simulink model "wiggler_frf_adxl"  (R2018a)
settings: Solver=FixedStepDiscrete  StartTime=0.0  StopTime=10.0  RelTol=1e-3
PreLoadFcn:
  | waijung.modelPreload; % Required for working with Waijung Blockset. Do not remove.
undefined symbols (not defined in the file or in its folder): HSEOSC, Link, LQFP144, ST, STM32F446ZE
libraries: commsynccomp2 x38, simulink x10, stm32f4_io_lib x3, dspstat3 x2, stm32f4_device_config_lib x1, dspbuff3 x1
(part 2 of 4)

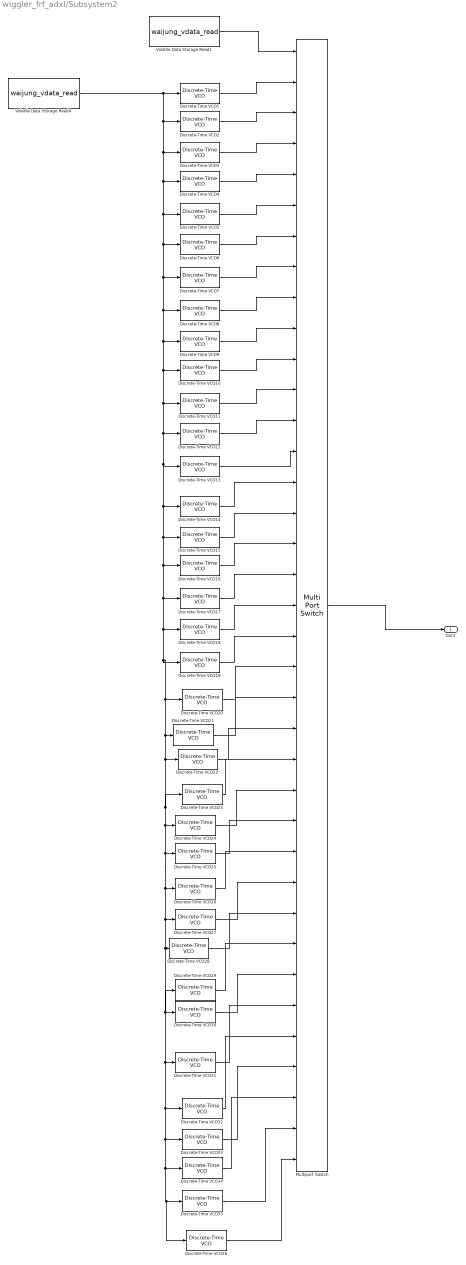
== system wiggler_frf_adxl/Subsystem2 ==
  Discrete-Time VCO1 : commsynccomp2/Discrete-Time VCO  Ac=1  Fc=0  Kc=1  Ph=0  ts=1e-3
      settings: SourceProductName=Communications System Toolbox  SourceProductBaseCode=CM
  Discrete-Time VCO10 : commsynccomp2/Discrete-Time VCO  Ac=1  Fc=0  Kc=1  Ph=(90/180)*pi  ts=1e-3
      settings: SourceProductName=Communications System Toolbox  SourceProductBaseCode=CM
  Discrete-Time VCO11 : commsynccomp2/Discrete-Time VCO  Ac=1  Fc=0  Kc=1  Ph=(100/180)*pi  ts=1e-3
      settings: SourceProductName=Communications System Toolbox  SourceProductBaseCode=CM
  Discrete-Time VCO12 : commsynccomp2/Discrete-Time VCO  Ac=1  Fc=0  Kc=1  Ph=(110/180)*pi  ts=1e-3
      settings: SourceProductName=Communications System Toolbox  SourceProductBaseCode=CM
  Discrete-Time VCO13 : commsynccomp2/Discrete-Time VCO  Ac=1  Fc=0  Kc=1  Ph=(120/180)*pi  ts=1e-3
      settings: SourceProductName=Communications System Toolbox  SourceProductBaseCode=CM
  Discrete-Time VCO14 : commsynccomp2/Discrete-Time VCO  Ac=1  Fc=0  Kc=1  Ph=(130/180)*pi  ts=1e-3
      settings: SourceProductName=Communications System Toolbox  SourceProductBaseCode=CM
  Discrete-Time VCO15 : commsynccomp2/Discrete-Time VCO  Ac=1  Fc=0  Kc=1  Ph=(140/180)*pi  ts=1e-3
      settings: SourceProductName=Communications System Toolbox  SourceProductBaseCode=CM
  Discrete-Time VCO16 : commsynccomp2/Discrete-Time VCO  Ac=1  Fc=0  Kc=1  Ph=(150/180)*pi  ts=1e-3
      settings: SourceProductName=Communications System Toolbox  SourceProductBaseCode=CM
  Discrete-Time VCO17 : commsynccomp2/Discrete-Time VCO  Ac=1  Fc=0  Kc=1  Ph=(160/180)*pi  ts=1e-3
      settings: SourceProductName=Communications System Toolbox  SourceProductBaseCode=CM
  Discrete-Time VCO18 : commsynccomp2/Discrete-Time VCO  Ac=1  Fc=0  Kc=1  Ph=(170/180)*pi  ts=1e-3
      settings: SourceProductName=Communications System Toolbox  SourceProductBaseCode=CM
  Discrete-Time VCO19 : commsynccomp2/Discrete-Time VCO  Ac=1  Fc=0  Kc=1  Ph=(180/180)*pi  ts=1e-3
      settings: SourceProductName=Communications System Toolbox  SourceProductBaseCode=CM
  Discrete-Time VCO2 : commsynccomp2/Discrete-Time VCO  Ac=1  Fc=0  Kc=1  Ph=(10/180)*pi  ts=1e-3
      settings: SourceProductName=Communications System Toolbox  SourceProductBaseCode=CM
  Discrete-Time VCO20 : commsynccomp2/Discrete-Time VCO  Ac=1  Fc=0  Kc=1  Ph=(190/180)*pi  ts=1e-3
      settings: SourceProductName=Communications System Toolbox  SourceProductBaseCode=CM
  Discrete-Time VCO21 : commsynccomp2/Discrete-Time VCO  Ac=1  Fc=0  Kc=1  Ph=(200/180)*pi  ts=1e-3
      settings: SourceProductName=Communications System Toolbox  SourceProductBaseCode=CM
  Discrete-Time VCO22 : commsynccomp2/Discrete-Time VCO  Ac=1  Fc=0  Kc=1  Ph=(210/180)*pi  ts=1e-3
      settings: SourceProductName=Communications System Toolbox  SourceProductBaseCode=CM
  Discrete-Time VCO23 : commsynccomp2/Discrete-Time VCO  Ac=1  Fc=0  Kc=1  Ph=(220/180)*pi  ts=1e-3
      settings: SourceProductName=Communications System Toolbox  SourceProductBaseCode=CM
  Discrete-Time VCO24 : commsynccomp2/Discrete-Time VCO  Ac=1  Fc=0  Kc=1  Ph=(230/180)*pi  ts=1e-3
      settings: SourceProductName=Communications System Toolbox  SourceProductBaseCode=CM
  Discrete-Time VCO25 : commsynccomp2/Discrete-Time VCO  Ac=1  Fc=0  Kc=1  Ph=(240/180)*pi  ts=1e-3
      settings: SourceProductName=Communications System Toolbox  SourceProductBaseCode=CM
  Discrete-Time VCO26 : commsynccomp2/Discrete-Time VCO  Ac=1  Fc=0  Kc=1  Ph=(250/180)*pi  ts=1e-3
      settings: SourceProductName=Communications System Toolbox  SourceProductBaseCode=CM
  Discrete-Time VCO27 : commsynccomp2/Discrete-Time VCO  Ac=1  Fc=0  Kc=1  Ph=(260/180)*pi  ts=1e-3
      settings: SourceProductName=Communications System Toolbox  SourceProductBaseCode=CM
  Discrete-Time VCO28 : commsynccomp2/Discrete-Time VCO  Ac=1  Fc=0  Kc=1  Ph=(270/180)*pi  ts=1e-3
      settings: SourceProductName=Communications System Toolbox  SourceProductBaseCode=CM
  Discrete-Time VCO29 : commsynccomp2/Discrete-Time VCO  Ac=1  Fc=0  Kc=1  Ph=(280/180)*pi  ts=1e-3
      settings: SourceProductName=Communications System Toolbox  SourceProductBaseCode=CM
  Discrete-Time VCO3 : commsynccomp2/Discrete-Time VCO  Ac=1  Fc=0  Kc=1  Ph=(20/180)*pi  ts=1e-3
      settings: SourceProductName=Communications System Toolbox  SourceProductBaseCode=CM
  Discrete-Time VCO30 : commsynccomp2/Discrete-Time VCO  Ac=1  Fc=0  Kc=1  Ph=(290/180)*pi  ts=1e-3
      settings: SourceProductName=Communications System Toolbox  SourceProductBaseCode=CM
  Discrete-Time VCO31 : commsynccomp2/Discrete-Time VCO  Ac=1  Fc=0  Kc=1  Ph=(300/180)*pi  ts=1e-3
      settings: SourceProductName=Communications System Toolbox  SourceProductBaseCode=CM
  Discrete-Time VCO32 : commsynccomp2/Discrete-Time VCO  Ac=1  Fc=0  Kc=1  Ph=(310/180)*pi  ts=1e-3
      settings: SourceProductName=Communications System Toolbox  SourceProductBaseCode=CM
  Discrete-Time VCO33 : commsynccomp2/Discrete-Time VCO  Ac=1  Fc=0  Kc=1  Ph=(320/180)*pi  ts=1e-3
      settings: SourceProductName=Communications System Toolbox  SourceProductBaseCode=CM
  Discrete-Time VCO34 : commsynccomp2/Discrete-Time VCO  Ac=1  Fc=0  Kc=1  Ph=(330/180)*pi  ts=1e-3
      settings: SourceProductName=Communications System Toolbox  SourceProductBaseCode=CM
  Discrete-Time VCO35 : commsynccomp2/Discrete-Time VCO  Ac=1  Fc=0  Kc=1  Ph=(340/180)*pi  ts=1e-3
      settings: SourceProductName=Communications System Toolbox  SourceProductBaseCode=CM
  Discrete-Time VCO36 : commsynccomp2/Discrete-Time VCO  Ac=1  Fc=0  Kc=1  Ph=(350/180)*pi  ts=1e-3
      settings: SourceProductName=Communications System Toolbox  SourceProductBaseCode=CM
  Discrete-Time VCO4 : commsynccomp2/Discrete-Time VCO  Ac=1  Fc=0  Kc=1  Ph=(30/180)*pi  ts=1e-3
      settings: SourceProductName=Communications System Toolbox  SourceProductBaseCode=CM
  Discrete-Time VCO5 : commsynccomp2/Discrete-Time VCO  Ac=1  Fc=0  Kc=1  Ph=(40/180)*pi  ts=1e-3
      settings: SourceProductName=Communications System Toolbox  SourceProductBaseCode=CM
  Discrete-Time VCO6 : commsynccomp2/Discrete-Time VCO  Ac=1  Fc=0  Kc=1  Ph=(50/180)*pi  ts=1e-3
      settings: SourceProductName=Communications System Toolbox  SourceProductBaseCode=CM
  Discrete-Time VCO7 : commsynccomp2/Discrete-Time VCO  Ac=1  Fc=0  Kc=1  Ph=(60/180)*pi  ts=1e-3
      settings: SourceProductName=Communications System Toolbox  SourceProductBaseCode=CM
  Discrete-Time VCO8 : commsynccomp2/Discrete-Time VCO  Ac=1  Fc=0  Kc=1  Ph=(70/180)*pi  ts=1e-3
      settings: SourceProductName=Communications System Toolbox  SourceProductBaseCode=CM
  Discrete-Time VCO9 : commsynccomp2/Discrete-Time VCO  Ac=1  Fc=0  Kc=1  Ph=(80/180)*pi  ts=1e-3
      settings: SourceProductName=Communications System Toolbox  SourceProductBaseCode=CM
  Multiport Switch : MultiPortSwitch  DataPortOrder=Zero-based contiguous  Inputs=36  zeroidx=on
  Volatile Data Storage Read1 : S-Function  FunctionName=waijung_vdata_read  Parameters=storagename,varname,sampletime,sampletimestr,blockid,storagetype,storagetypestr  SFunctionDeploymentMode=off  EnableBusSupport=off  mask(waijung_vdata_read){storagename=Phase, varname=VolatileDataStorage7_Phase, sampletime=.001, sampletimestr=-1, blockid=Subsystem2VolatileDataStorageRead1, storagetype=double, storagetypestr=double}
      mask prompts: storagename "Storage Name"; varname "Variable name"; sampletime "Sample time (sec)"; sampletimestr "Compiled sample time (sec) in string"; storagetype "Data type"; storagetypestr "Data type string"
      mask help: This block implements read data from a buffer.
      mask init:
      | waijung_vdata_read_callback('init');
      mask Help: web(fullfile(waijungdocroot,'Volatile_Data_Storage_Read.htm'))
      mask TypeOptions storagename: Laser | Ax | flag | fx | fy | Ay | Phase
      mask Callback storagename: waijung_vdata_read_callback('storagename');
      mask Callback varname: waijung_vdata_read_callback('varname');
      mask Callback sampletime: waijung_vdata_read_callback('sampletime');
      mask Callback sampletimestr: waijung_vdata_read_callback('sampletimestr');
      mask Callback blockid: waijung_vdata_read_callback('blockid');
      mask Callback storagetype: waijung_vdata_read_callback('storagetype');
      mask Display: text(0.05, 0.5, 'Buffer: Phase','ver','middle','hor','left');port_label('output',1,'D1(double)')
  Volatile Data Storage Read4 : S-Function  FunctionName=waijung_vdata_read  Parameters=storagename,varname,sampletime,sampletimestr,blockid,storagetype,storagetypestr  SFunctionDeploymentMode=off  EnableBusSupport=off  mask(waijung_vdata_read){storagename=fy, varname=VolatileDataStorage5_fy, sampletime=.001, sampletimestr=-1, blockid=Subsystem2VolatileDataStorageRead4, storagetype=double, storagetypestr=double}
      mask prompts: storagename "Storage Name"; varname "Variable name"; sampletime "Sample time (sec)"; sampletimestr "Compiled sample time (sec) in string"; storagetype "Data type"; storagetypestr "Data type string"
      mask help: This block implements read data from a buffer.
      mask init:
      | waijung_vdata_read_callback('init');
      mask Help: web(fullfile(waijungdocroot,'Volatile_Data_Storage_Read.htm'))
      mask TypeOptions storagename: Laser | Ax | flag | fx | fy | Ay | Phase
      mask Callback storagename: waijung_vdata_read_callback('storagename');
      mask Callback varname: waijung_vdata_read_callback('varname');
      mask Callback sampletime: waijung_vdata_read_callback('sampletime');
      mask Callback sampletimestr: waijung_vdata_read_callback('sampletimestr');
      mask Callback blockid: waijung_vdata_read_callback('blockid');
      mask Callback storagetype: waijung_vdata_read_callback('storagetype');
      mask Display: text(0.05, 0.5, 'Buffer: fy','ver','middle','hor','left');port_label('output',1,'D1(double)')
  Out2 : Outport
  wires:
  Volatile Data Storage Read4/1 -> Discrete-Time VCO36/1, Discrete-Time VCO35/1, Discrete-Time VCO34/1, Discrete-Time VCO33/1, Discrete-Time VCO32/1, Discrete-Time VCO31/1, Discrete-Time VCO30/1, Discrete-Time VCO29/1, Discrete-Time VCO28/1, Discrete-Time VCO27/1, Discrete-Time VCO26/1, Discrete-Time VCO25/1, Discrete-Time VCO24/1, Discrete-Time VCO23/1, Discrete-Time VCO22/1, Discrete-Time VCO21/1, Discrete-Time VCO20/1, Discrete-Time VCO19/1, Discrete-Time VCO18/1, Discrete-Time VCO17/1, Discrete-Time VCO16/1, Discrete-Time VCO15/1, Discrete-Time VCO14/1, Discrete-Time VCO13/1, Discrete-Time VCO12/1, Discrete-Time VCO11/1, Discrete-Time VCO10/1, Discrete-Time VCO9/1, Discrete-Time VCO8/1, Discrete-Time VCO7/1, Discrete-Time VCO6/1, Discrete-Time VCO5/1, Discrete-Time VCO4/1, Discrete-Time VCO3/1, Discrete-Time VCO2/1, Discrete-Time VCO1/1
  Discrete-Time VCO1/1 -> Multiport Switch/2
  Discrete-Time VCO2/1 -> Multiport Switch/3
  Discrete-Time VCO3/1 -> Multiport Switch/4
  Discrete-Time VCO4/1 -> Multiport Switch/5
  Discrete-Time VCO5/1 -> Multiport Switch/6
  Discrete-Time VCO6/1 -> Multiport Switch/7
  Discrete-Time VCO7/1 -> Multiport Switch/8
  Discrete-Time VCO8/1 -> Multiport Switch/9
  Discrete-Time VCO9/1 -> Multiport Switch/10
  Discrete-Time VCO10/1 -> Multiport Switch/11
  Discrete-Time VCO11/1 -> Multiport Switch/12
  Discrete-Time VCO12/1 -> Multiport Switch/13
  Discrete-Time VCO13/1 -> Multiport Switch/14
  Discrete-Time VCO14/1 -> Multiport Switch/15
  Discrete-Time VCO15/1 -> Multiport Switch/16
  Discrete-Time VCO16/1 -> Multiport Switch/17
  Discrete-Time VCO17/1 -> Multiport Switch/18
  Discrete-Time VCO18/1 -> Multiport Switch/19
  Discrete-Time VCO19/1 -> Multiport Switch/20
  Discrete-Time VCO20/1 -> Multiport Switch/21
  Discrete-Time VCO21/1 -> Multiport Switch/22
  Discrete-Time VCO22/1 -> Multiport Switch/23
  Discrete-Time VCO23/1 -> Multiport Switch/24
  Discrete-Time VCO24/1 -> Multiport Switch/25
  Discrete-Time VCO25/1 -> Multiport Switch/26
  Discrete-Time VCO26/1 -> Multiport Switch/27
  Discrete-Time VCO27/1 -> Multiport Switch/28
  Discrete-Time VCO28/1 -> Multiport Switch/29
  Discrete-Time VCO29/1 -> Multiport Switch/30
  Discrete-Time VCO30/1 -> Multiport Switch/31
  Discrete-Time VCO31/1 -> Multiport Switch/32
  Discrete-Time VCO32/1 -> Multiport Switch/33
  Discrete-Time VCO33/1 -> Multiport Switch/34
  Discrete-Time VCO34/1 -> Multiport Switch/35
  Discrete-Time VCO35/1 -> Multiport Switch/36
  Discrete-Time VCO36/1 -> Multiport Switch/37
  Multiport Switch/1 -> Out2/1
  Volatile Data Storage Read1/1 -> Multiport Switch/1

== system wiggler_frf_adxl/UART_parameter_input ==

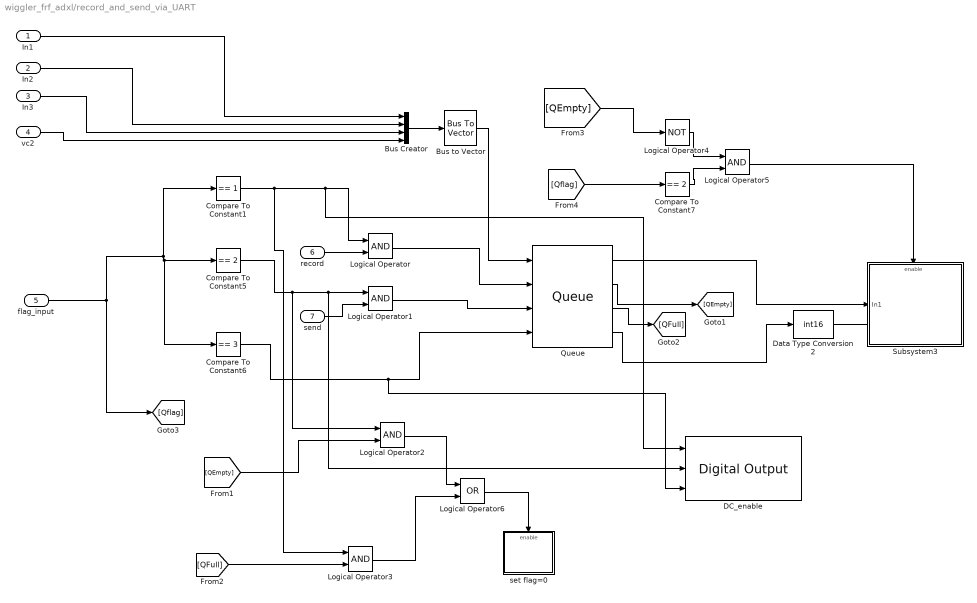
== system wiggler_frf_adxl/record_and_send_via_UART ==
  In1 : Inport
  In2 : Inport  Port=2
  In3 : Inport  Port=3
  vc2 : Inport  Port=4
  flag_input : Inport  Port=5
  record : Inport  Port=6
  send : Inport  Port=7
  Bus Creator : BusCreator  Inputs=4
  Bus to Vector : BusToVector
  Compare To Constant1 : simulink/Logic and Bit Operations/Compare To Constant  relop===  const=1  OutDataTypeStr=boolean
  Compare To Constant5 : simulink/Logic and Bit Operations/Compare To Constant  relop===  const=2  OutDataTypeStr=boolean
  Compare To Constant6 : simulink/Logic and Bit Operations/Compare To Constant  relop===  const=3  OutDataTypeStr=boolean
  Compare To Constant7 : simulink/Logic and Bit Operations/Compare To Constant  relop===  const=2  OutDataTypeStr=boolean
  DC_enable : stm32f4_io_lib/Digital Output  use_bitband=on  port=B  speed=100  porttype=Push Pull  porttypestr=PP  use_pin0=on  use_pin1=off  use_pin2=off  use_pin3=off  use_pin4=off  use_pin5=off  use_pin6=off  use_pin7=on  use_pin8=off  use_pin9=off  use_pin10=off  use_pin11=off  use_pin12=off  use_pin13=off  use_pin14=on  use_pin15=off  pinstr=GPIO_Pin_0 | GPIO_Pin_7 | GPIO_Pin_14  usedpinarray="[1  0  0  0  0  0  0  1  0  0  0  0  0  0  1  0]"  bitbandingstr=|  sampletime=-1  sampletimestr=-1  blockid=record_and_send_via_UARTDC_enable  enablecustomportlabel=off  globalinit=off  cinputportlabel=In1, In2  coutputportlabel=0
      | #define record_and_send_via_UARTDC_enable_B0 Peripheral_BB(GPIOB->ODR, 0)  /* Output pin */
      | #define record_and_send_via_UARTDC_enable_B7 Peripheral_BB(GPIOB->ODR, 7)  /* Output pin */
      | #define record_and_send_via_UARTDC_enable_B14 Peripheral_BB(GPIOB->ODR, 14)  /* Output pin */
      settings: SourceProductName=Waijung Blockset
  Data Type Conversion2 : DataTypeConversion  OutDataTypeStr=int16
  Logical Operator{,1..3,5} (5 alike) : Logic  AllPortsSameDT=off  OutDataTypeStr=boolean
  Logical Operator4 : Logic  Operator=NOT  AllPortsSameDT=off  OutDataTypeStr=boolean
  Logical Operator6 : Logic  Operator=OR  AllPortsSameDT=off  OutDataTypeStr=boolean
  Queue : dspbuff3/Queue  depth=3000  trigger=Either edge  overflow=Ignore  pes=Ignore  eso=on  fso=on  nso=on  clr=on  clrOutport=on  adf=on
      settings: SourceProductName=DSP System Toolbox  SourceProductBaseCode=DS
  Subsystem3 : Subsystem
  set flag=0 : Subsystem
  wires:
  send/1 -> Logical Operator1/2
  [QFull] -> Logical Operator3/2
  Queue/4 -> Data Type Conversion2/1
  Logical Operator/1 -> Queue/2
  record/1 -> Logical Operator/2
  Logical Operator1/1 -> Queue/3
  Queue/2 -> [QEmpty]
  Logical Operator3/1 -> Logical Operator6/2
  Compare To Constant7/1 -> Logical Operator5/2
  Compare To Constant5/1 -> DC_enable/2, Logical Operator1/1, Logical Operator2/1
  Compare To Constant1/1 -> Logical Operator3/1, DC_enable/1, Logical Operator/1
  [QEmpty] -> Logical Operator2/2
  Compare To Constant6/1 -> DC_enable/3, Queue/4
  [QEmpty] -> Logical Operator4/1
  Logical Operator4/1 -> Logical Operator5/1
  Queue/3 -> [QFull]
  [Qflag] -> Compare To Constant7/1
  Logical Operator5/1 -> Subsystem3/Enable
  Logical Operator6/1 -> set flag=0/Enable
  Bus Creator/1 -> Bus to Vector/1
  Bus to Vector/1 -> Queue/1
  In2/1 -> Bus Creator/2
  Logical Operator2/1 -> Logical Operator6/1
  In1/1 -> Bus Creator/1
  Queue/1 -> Subsystem3/1(In1)
  flag_input/1 -> [Qflag], Compare To Constant6/1, Compare To Constant5/1, Compare To Constant1/1
  Data Type Conversion2/1 -> ?
  In3/1 -> Bus Creator/3
  vc2/1 -> Bus Creator/4
